simulink model "AE426SIMULINK8_2UnrealEditor"  (R2024b)
settings: Solver=ode4  StartTime=0  StopTime=simlength  FixedStep=dt  RelTol=1e-3
InitFcn:
  | clear
  | clf
  | close all
  | wrlFilePath = fullfile(pwd, 'SpacecraftEarth.wrl');
  | myworld = vrworld(wrlFilePath);
  | open(myworld);
  | set(0,'Units','pixels');
  | 
  | screenSize = get(0, 'ScreenSize');
  | screenWidth = screenSize(3);
  | screenHeight = screenSize(4);
  | figWidth = screenWidth / 3;
  | figHeight = screenHeight / 2;
  | 
  | positions = [
  |      screenHeight - figHeight, 0, figWidth, figHeight; % Top-left
  |      figWidth, screenHeight - figHeight, figWidth, figHeight; % Top-right
  |      2*figWidth, screenHeight - figHeight, figWidth, figHeight; % Bottom-left
  | ];
  | 
  | %fig1 = vrfigure(myworld,positions(1, :));
  | %set(fig1,'Viewpoint','WorldView');
  | 
  | %fig2 = vrfigure(myworld,positions(2, :));
  | %set(fig2,'Viewpoint','NadirView');
  | 
  | %fig3 = vrfigure(myworld,positions(3, :));
  | %set(fig3,'Viewpoint','TargetView');
  | 
  | %vrsetpref DefaultFigurePlaneClipMethod bvolume
  | 
  | mu = 3.986004e5;
  | dt = 0.01;
  | % ypr0 = [pi/4,pi/6,-pi/6];
  | % q1 = sin(ypr0(3)/2)*cos(ypr0(2)/2)*cos(ypr0(1)/2)-cos(ypr0(3)/2)*sin(ypr0(2)/2)*sin(ypr0(1)/2);
  | % q2 = sin(ypr0(3)/2)*cos(ypr0(2)/2)*sin(ypr0(1)/2)+cos(ypr0(3)/2)*sin(ypr0(2)/2)*cos(ypr0(1)/2);
  | % q3 = cos(ypr0(3)/2)*cos(ypr0(2)/2)*sin(ypr0(1)/2)-sin(ypr0(3)/2)*sin(ypr0(2)/2)*cos(ypr0(1)/2);
  | % q4 = cos(ypr0(3)/2)*cos(ypr0(2)/2)*cos(ypr0(1)/2)+sin(ypr0(3)/2)*sin(ypr0(2)/2)*sin(ypr0(1)/2);
  | % q0 = [q1;q2;q3;q4];
  | q0 = [0;0;0;1];
  | w0 = [0.000;0.000;0.000];
  | H0 = [0;0;0];
  | lat = [34.6178 34.9438 34.3658].*pi./180;
  | long = [-112.4503 -111.7529 -111.4481].*pi./180;
  | longlat = [long;lat]';
  | % Earth's equatorial radius
  | a = 6378.137;
  | % Earth's eccentricity
  | e = 0.08181919;
  | % Latitude (radians)
  | phi = deg2rad(34.54002);
  | % Longitude (radians)
  | lambda = deg2rad(-112.4685);
  | % Earth's rotation rate (rad/s)
  | omega = (2 *pi)/86164;
  | % Altitude (km)
  | h = 36.5;
  | 
  | % Compute Earth's radius at latitude (WGS-84)
  | Rn = a / sqrt(1 - (e^2 * sin(phi)^2));
  | ... (+59 lines)
StopFcn:
  | %/*data = get(out,"YPR");
  | %data_e1 = get(out,"TargetYPR");
  | %t = data.time - 51744.4;
  | 
  | %y = data.Data(:,1);
  | %p = data.Data(:,2);
  | %r = data.Data(:,3);
  | %ye = data_e1.Data(:,1);
  | %pe = data_e1.Data(:,2);
  | %re = data_e1.Data(:,3);
  | %figure(1);
  | 
  | %subplot(1,3,1);
  | %hold on
  | %plot(t, y*180/pi, 'b')
  | %plot(t, ye*180/pi, '--r')
  | %hold off
  | %ylabel('Yaw (deg)')
  | %xlabel('Time (s)')
  | %grid on
  | 
  | %subplot(1,3,2);
  | %hold on
  | %plot(t, p*180/pi, 'b')
  | %plot(t, pe*180/pi, '--r')
  | %hold off
  | %ylabel('Pitch (deg)')
  | %xlabel('Time (s)')
  | %grid on
  | 
  | %subplot(1,3,3);
  | %hold on
  | %plot(t, r*180/pi, 'b')
  | %plot(t, re*180/pi, '--r')
  | %hold off
  | %ylabel('Roll (deg)')
  | %xlabel('Time (s)')
  | %grid on
  | 
  | %data2 = get(out,"Torque");
  | %t = data2.time - 51744.4;
  | 
  | %y = data2.Data(3,:);
  | %p = data2.Data(2,:);
  | %r = data2.Data(1,:);
  | %figure(2);
  | %subplot(1,3,1);
  | %plot(t, y, 'b')
  | %ylabel('T_Y (N*m)')
  | %xlabel('Time (s)')
  | %grid on
  | %subplot(1,3,2);
  | %plot(t, p, 'b')
  | %ylabel('T_P (N*m)')
  | %xlabel('Time (s)')
  | %grid on
  | %subplot(1,3,3);
  | %plot(t, r, 'b')
  | %ylabel('T_R (N*m)')
  | %xlabel('Time (s)')
  | ... (+23 lines)
undefined symbols (not defined in the file): gray, K, Sim3dSensor
libraries: matrix_library x9, vrlib x7, sim3dlib x5, simulink x1
(part 2 of 2)

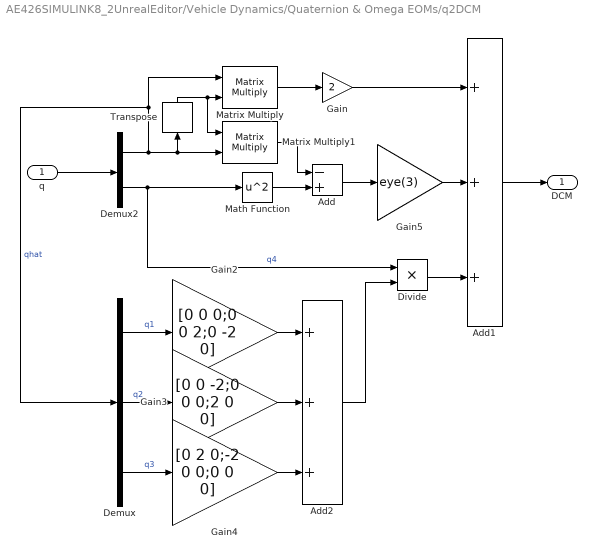
== system AE426SIMULINK8_2UnrealEditor/Vehicle Dynamics/Quaternion & Omega EOMs/q2DCM ==
  q : Inport
  Add : Sum  Inputs=-+
  Add1 : Sum  Inputs=+++
  Add2 : Sum  Inputs=+++
  Demux : Demux  Outputs=3
  Demux2 : Demux  Outputs=[3,1]
  Divide : Product  Inputs=**
  Gain : Gain  Gain=2
  Gain2 : Gain  Gain=[0 0 0;0 0 2;0 -2 0]
  Gain3 : Gain  Gain=[0 0 -2;0 0 0;2 0 0]
  Gain4 : Gain  Gain=[0 2 0;-2 0 0;0 0 0]
  Gain5 : Gain  Gain=eye(3)
  Math Function : Math  Operator=square
  Matrix Multiply : Product  Multiplication=Matrix(*)
  Matrix Multiply1 : Product  Multiplication=Matrix(*)
  Transpose : matrix_library/Transpose
  DCM : Outport
  wires:
  Math Function/1 -> Add/2
  Matrix Multiply1/1 -> Add/1
  Add2/1 -> Divide/2
  Gain/1 -> Add1/1
  Transpose/1 -> Matrix Multiply1/1, Matrix Multiply/2
  Demux/2 -> Gain3/1  "q2"
  Gain3/1 -> Add2/2
  Demux2/2 -> Divide/1, Math Function/1  "q4"
  Matrix Multiply/1 -> Gain/1
  Demux/1 -> Gain2/1  "q1"
  Gain5/1 -> Add1/2
  Divide/1 -> Add1/3
  Gain2/1 -> Add2/1
  Demux/3 -> Gain4/1  "q3"
  Gain4/1 -> Add2/3
  Add/1 -> Gain5/1
  Demux2/1 -> Matrix Multiply1/2, Transpose/1, Matrix Multiply/1, Demux/1  "qhat"
  q/1 -> Demux2/1
  Add1/1 -> DCM/1

== system AE426SIMULINK8_2UnrealEditor/Vehicle Dynamics/Quaternion & Omega EOMs/thetas ==
  r : Inport
  v : Inport  Port=2
  Cross Product1 : matrix_library/Cross Product
  Divide : Product  Inputs=/*
  Divide1 : Product  Inputs=*/*
  Dot Product : DotProduct  OutDataTypeStr=Inherit: Inherit via internal rule
  Dot Product1 : DotProduct  OutDataTypeStr=Inherit: Inherit via internal rule
  Dot Product2 : DotProduct  OutDataTypeStr=Inherit: Inherit via internal rule
  Gain3 : Gain  Gain=[0;-1;0]
  Gain4 : Gain  Gain=-2
  Sqrt : Sqrt
  -theta double dot : Outport
  -theta dot : Outport  Port=2
  wires:
  Divide/1 -> Gain3/1  "theta dot"
  Dot Product/1 -> Sqrt/1
  v/1 -> Cross Product1/2, Dot Product2/1
  Dot Product1/1 -> Divide1/2, Divide/1  "r^2"
  Gain3/1 -> -theta dot/1, Divide1/3  "-theta dot"
  Divide1/1 -> Gain4/1
  Cross Product1/1 -> Dot Product/1, Dot Product/2
  r/1 -> Cross Product1/1, Dot Product1/1, Dot Product1/2, Dot Product2/2
  Sqrt/1 -> Divide/2
  Dot Product2/1 -> Divide1/1
  Gain4/1 -> -theta double dot/1  "-theta double dot"
